simulink model "SADS_UKF"  (R2024b)
settings: Solver=ode15s  StartTime=0.0  StopTime=t_final  RelTol=1e-3
values from neighbouring files (symbols this model uses):
  EA_0 = deg2rad(output(2:4,1))    [telemetry.m]
  g_N = [0 0 -9.81]    [telemetry.m]
  H = [eye(3)  zeros(3,5)]    [telemetry.m]
  J = [1.301  0 0 ... (first row only)    [playground.m]    (also in telemetry.m)
  m_s = 28.542    [playground.m]    (also in telemetry.m)
  omega_0 = output(5:7,1)    [telemetry.m]
  P_0 = diag([1e-6 1e-6 1e-6 1e-6 1e-6 1e-6 1e-6 1e-6])    [telemetry.m]
  process_PSD = (process_variance^2)*T_s    (= 1e-12)    [telemetry.m]
  Q = diag([5e-5 5e-5 5e-5 4e-11 4e-11 4e-11 4e-11 4e-13])    [telemetry.m]
  q_0 = eul2quat(EA_0',"XYZ")'    [telemetry.m]
  R = diag([0.005 0.005 0.003].^2)    [telemetry.m]
  r_0 = [-0.003 0.006 -0.005]'    [telemetry.m]
  sample_time = 1/sample_rate    (= 0.04)    [telemetry.m]
  sensor_PSD = noise_power^2    (= 2.74155703361e-09)    [telemetry.m]
  x_0 = [omega_0; q_0; -0.001]    [telemetry.m]
libraries: simulink x6, sharedtransform x2, simulink_extras x1
settings Model: Creator=camer  LastModifiedBy=camer

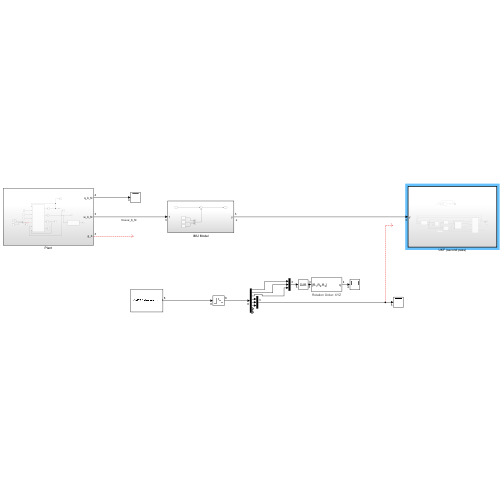
[thumbnail: Simulink's stored preview of the top-level diagram]
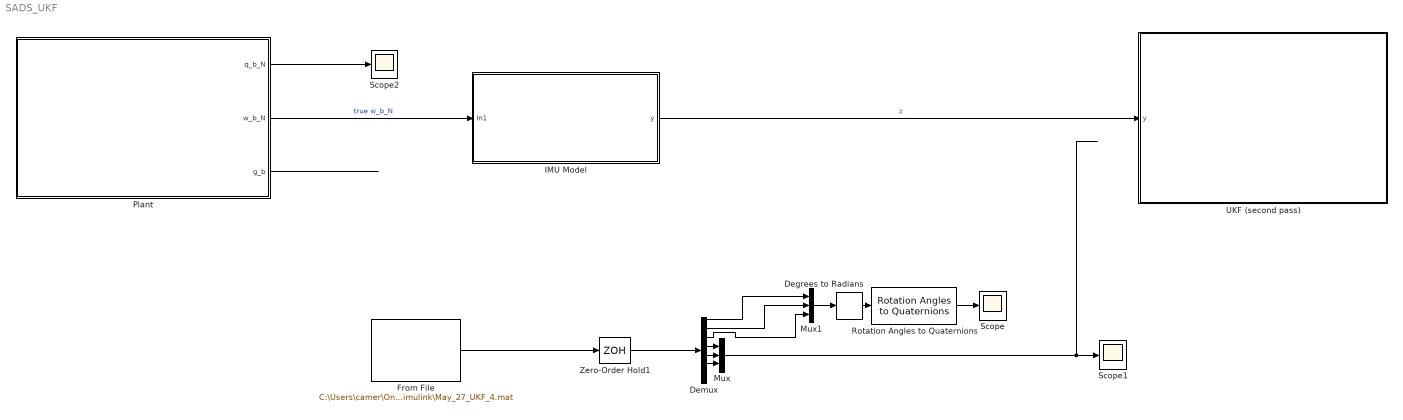
== system SADS_UKF ==
  Degrees to Radians : simulink_extras/Transformations/Degrees to Radians
  Demux : Demux  Outputs=8
  From File : FromFile  FileName=C:\Users\camer\OneDrive\Desktop\SADS Balance\export_for_simulink\May_27_UKF_4.mat  SampleTime=0  InterpolationWithinTimeRange=Zero order hold
  IMU Model : Subsystem
  Mux : Mux  Inputs=3
  Mux1 : Mux  Inputs=3
  Plant : Subsystem
  Rotation Angles to Quaternions : sharedtransform/Rotation Angles to Quaternions  rotationOrder=XYZ  aMode=aMode
  Scope : Scope
  Scope1 : Scope
  Scope2 : Scope
  UKF (second pass) : Subsystem  TreatAsAtomicUnit=on
  Zero-Order Hold1 : ZeroOrderHold  SampleTime=sample_time
  wires:
  Plant/2(w_b_N) -> IMU Model/1(In1)  "true w_b_N"
  Plant/3(g_b) -> ?
  Plant/1(q_b_N) -> Scope2/1
  IMU Model/1(y) -> UKF (second pass)/1(y)  "z"
  Mux/1 -> Scope1/1
  From File/1 -> Zero-Order Hold1/1
  Zero-Order Hold1/1 -> Demux/1
  Demux/4 -> Mux/1
  Demux/5 -> Mux/2
  Demux/6 -> Mux/3
  Demux/1 -> Mux1/1
  Demux/2 -> Mux1/2
  Demux/3 -> Mux1/3
  Mux1/1 -> Degrees to Radians/1
  Degrees to Radians/1 -> Rotation Angles to Quaternions/1
  Rotation Angles to Quaternions/1 -> Scope/1

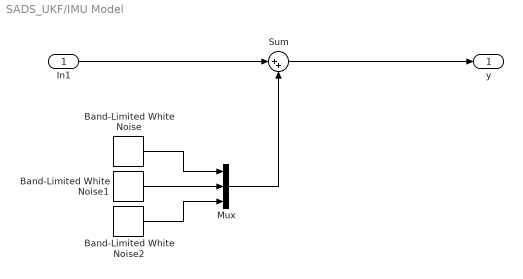
== system SADS_UKF/IMU Model ==
  In1 : Inport
  Band-Limited White Noise : simulink/Sources/Band-Limited White Noise  Cov=[sensor_PSD]  Ts=sample_time  seed=[23341]
  Band-Limited White Noise1 : simulink/Sources/Band-Limited White Noise  Cov=[sensor_PSD]  Ts=sample_time  seed=[23141]
  Band-Limited White Noise2 : simulink/Sources/Band-Limited White Noise  Cov=[sensor_PSD]  Ts=sample_time  seed=[35163]
  Mux : Mux  Inputs=3
  Sum : Sum  Inputs=|++
  y : Outport
  wires:
  Band-Limited White Noise1/1 -> Mux/2
  Band-Limited White Noise/1 -> Mux/1
  Band-Limited White Noise2/1 -> Mux/3
  In1/1 -> Sum/1
  Mux/1 -> Sum/2
  Sum/1 -> y/1

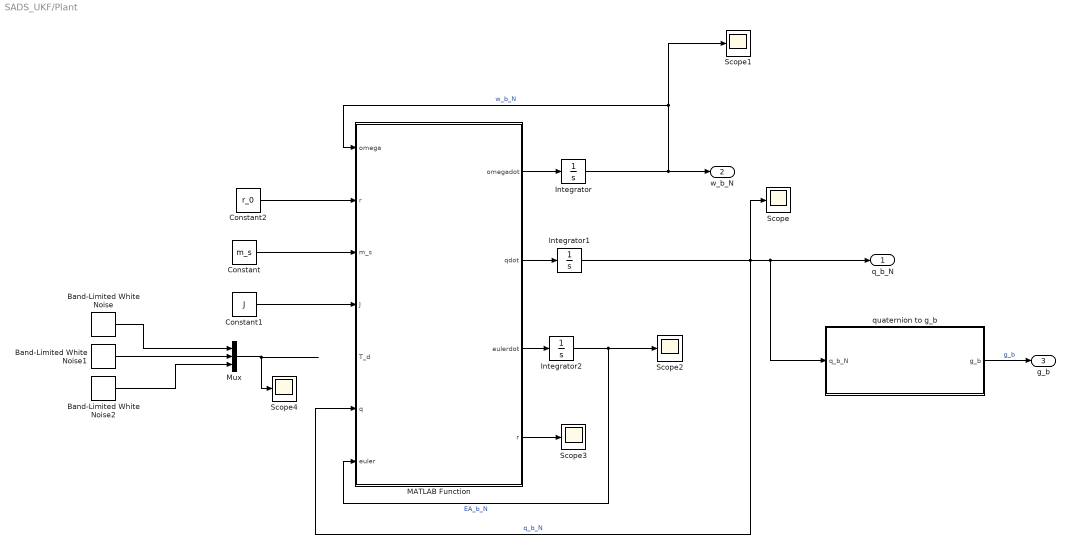
== system SADS_UKF/Plant ==
  Band-Limited White Noise : simulink/Sources/Band-Limited White Noise  Cov=[process_PSD]  Ts=0.1  seed=[23341]
  Band-Limited White Noise1 : simulink/Sources/Band-Limited White Noise  Cov=[process_PSD]  Ts=0.1  seed=[56123]
  Band-Limited White Noise2 : simulink/Sources/Band-Limited White Noise  Cov=[process_PSD]  Ts=0.1  seed=[31256]
  Constant : Constant  Value=m_s
  Constant1 : Constant  Value=J
  Constant2 : Constant  Value=r_0
  Integrator : Integrator  InitialCondition=omega_0
  Integrator1 : Integrator  InitialCondition=q_0
  Integrator2 : Integrator  InitialCondition=EA_0
  MATLAB Function : MATLAB Function  TreatAsAtomicUnit=on
  Mux : Mux  Inputs=3
  Scope{,1..4} (5 alike) : Scope
  quaternion to g_b : Subsystem
  q_b_N : Outport
  w_b_N : Outport  Port=2
  g_b : Outport  Port=3
  wires:
  MATLAB Function/4(r) -> Scope3/1
  Integrator/1 -> Scope1/1, MATLAB Function/1(omega), w_b_N/1  "w_b_N"
  Constant1/1 -> MATLAB Function/4(J)
  Constant2/1 -> MATLAB Function/2("r ")
  Constant/1 -> MATLAB Function/3(m_s)
  Integrator1/1 -> Scope/1, quaternion to g_b/1(q_b_N), q_b_N/1, MATLAB Function/6(q)  "q_b_N"
  MATLAB Function/2(qdot) -> Integrator1/1
  MATLAB Function/1(omegadot) -> Integrator/1
  quaternion to g_b/1(g_b) -> g_b/1  "g_b"
  MATLAB Function/3(eulerdot) -> Integrator2/1
  Integrator2/1 -> Scope2/1, MATLAB Function/7(euler)  "EA_b_N"
  Band-Limited White Noise/1 -> Mux/1
  Band-Limited White Noise1/1 -> Mux/2
  Band-Limited White Noise2/1 -> Mux/3
  Mux/1 -> Scope4/1

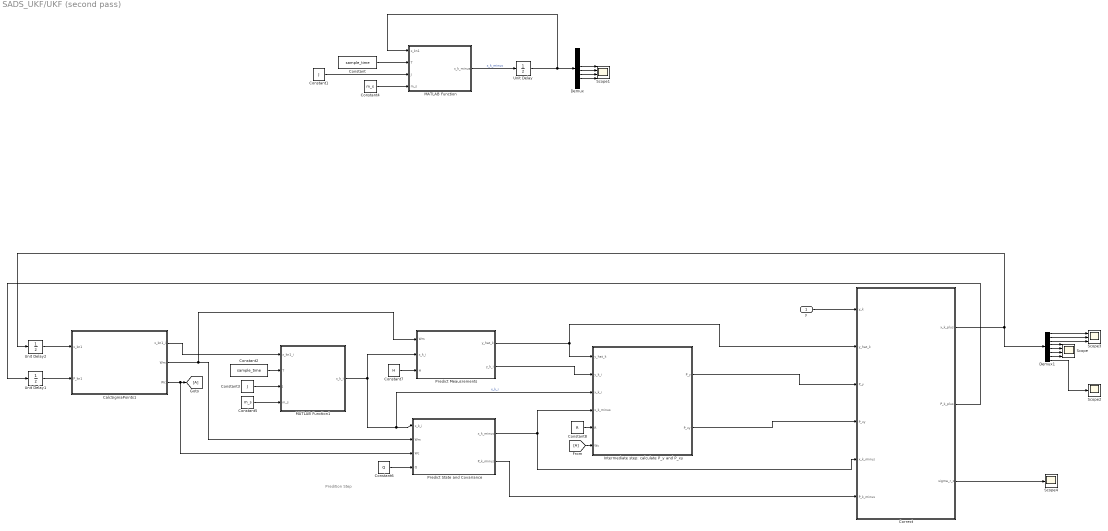
== system SADS_UKF/UKF (second pass) ==
  note: Predition Step
  y : Inport
  CalcSigmaPoints1 : MATLAB Function  TreatAsAtomicUnit=on
  Constant : Constant  Value=sample_time
  Constant1 : Constant  Value=J
  Constant2 : Constant  Value=sample_time
  Constant3 : Constant  Value=J
  Constant4 : Constant  Value=m_s
  Constant5 : Constant  Value=m_s
  Constant6 : Constant  Value=Q
  Constant7 : Constant  Value=H
  Constant8 : Constant  Value=R
  Correct : MATLAB Function  TreatAsAtomicUnit=on
  Demux : Demux  Outputs=8
  Demux1 : Demux  Outputs=8
  From : From
  Goto : Goto
  Intermediate step: calculate P_y and P_xy : MATLAB Function  TreatAsAtomicUnit=on
  MATLAB Function : MATLAB Function  TreatAsAtomicUnit=on
  MATLAB Function1 : MATLAB Function  TreatAsAtomicUnit=on
  Predict Meausrements : MATLAB Function  TreatAsAtomicUnit=on
  Predict State and Covariance : MATLAB Function  TreatAsAtomicUnit=on
  Scope : Scope  NumInputPorts=4
  Scope1 : Scope  NumInputPorts=4
  Scope2 : Scope
  Scope3 : Scope  NumInputPorts=3
  Scope4 : Scope
  Unit Delay : UnitDelay  InitialCondition=x_0  SampleTime=sample_time  HasFrameUpgradeWarning=on
  Unit Delay1 : UnitDelay  InitialCondition=P_0  SampleTime=sample_time  HasFrameUpgradeWarning=on
  Unit Delay2 : UnitDelay  InitialCondition=x_0  SampleTime=sample_time  HasFrameUpgradeWarning=on
  wires:
  MATLAB Function/1(x_k_minus) -> Unit Delay/1  "x_k_minus"
  Constant/1 -> MATLAB Function/2(T)
  Unit Delay/1 -> Demux/1, MATLAB Function/1(x_kn1)
  Constant1/1 -> MATLAB Function/3(J)
  CalcSigmaPoints1/1(x_kn1_i) -> MATLAB Function1/1(x_kn1_i)
  Constant3/1 -> MATLAB Function1/3(J)
  Constant2/1 -> MATLAB Function1/2(T)
  MATLAB Function1/1(x_k_i) -> Intermediate step: calculate P_y and P_xy/3(x_k_i), Predict State and Covariance/1(x_k_i), Predict Meausrements/2(x_k_i)  "x_k_i"
  Constant6/1 -> Predict State and Covariance/4(Q)
  Predict State and Covariance/1(x_k_minus) -> Intermediate step: calculate P_y and P_xy/4(x_k_minus), Correct/5(x_k_minus)
  Predict Meausrements/1(y_hat_k) -> Intermediate step: calculate P_y and P_xy/1(y_hat_k), Correct/2(y_hat_k)
  Predict State and Covariance/2(P_k_minus) -> Correct/6(P_k_minus)
  Constant7/1 -> Predict Meausrements/3(H)
  Predict Meausrements/2(y_k_i) -> Intermediate step: calculate P_y and P_xy/2(y_k_i)
  Constant8/1 -> Intermediate step: calculate P_y and P_xy/5(R)
  y/1 -> Correct/1(y_k)
  Intermediate step: calculate P_y and P_xy/1(P_y) -> Correct/3(P_y)
  Intermediate step: calculate P_y and P_xy/2(P_xy) -> Correct/4(P_xy)
  Correct/2(P_k_plus) -> Unit Delay1/1
  Correct/1(x_k_plus) -> Demux1/1, Unit Delay2/1
  Unit Delay1/1 -> CalcSigmaPoints1/2(P_kn1)
  Unit Delay2/1 -> CalcSigmaPoints1/1(x_kn1)
  CalcSigmaPoints1/2(Wm) -> Predict State and Covariance/2(Wm), Predict Meausrements/1(Wm)
  CalcSigmaPoints1/3(Wc) -> Goto/1, Predict State and Covariance/3(Wc)
  From/1 -> Intermediate step: calculate P_y and P_xy/6(Wc)
  Constant4/1 -> MATLAB Function/4(m_s)
  Demux/4 -> Scope1/1
  Demux/5 -> Scope1/2
  Demux/6 -> Scope1/3
  Demux/7 -> Scope1/4
  Demux1/5 -> Scope/2
  Demux1/4 -> Scope/1
  Demux1/6 -> Scope/3
  Demux1/7 -> Scope/4
  Constant5/1 -> MATLAB Function1/4(m_s)
  Demux1/8 -> Scope2/1
  Demux1/1 -> Scope3/1
  Demux1/2 -> Scope3/2
  Demux1/3 -> Scope3/3
  Correct/3(sigma_r_z) -> Scope4/1

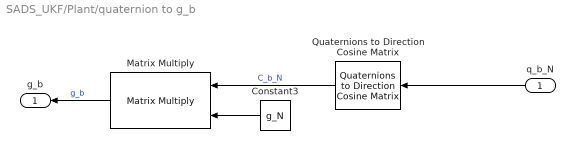
== system SADS_UKF/Plant/quaternion to g_b ==
  q_b_N : Inport
  Constant3 : Constant  Value=g_N
  Matrix Multiply : Product  Multiplication=Matrix(*)
  Quaternions to Direction Cosine Matrix : sharedtransform/Quaternions to  Direction Cosine Matrix  aMode=aMode
  g_b : Outport
  wires:
  Constant3/1 -> Matrix Multiply/2
  Quaternions to Direction Cosine Matrix/1 -> Matrix Multiply/1  "C_b_N"
  q_b_N/1 -> Quaternions to Direction Cosine Matrix/1
  Matrix Multiply/1 -> g_b/1  "g_b"

== matlab function SADS_UKF/UKF (second pass)/Predict State and Covariance ==
  data: x_k_i input; Wm input; Wc input; x_k_minus output; P_k_minus output; Q input
function [x_k_minus,P_k_minus] = predict_state_and_covariance(x_k_i,Wm,Wc,Q)

x_k_minus = x_k_i * Wm;  % weighted mean  (matrix‑vector product)
x_k_minus(4:7) = x_k_minus(4:7)./norm(x_k_minus(4:7));

P_k_minus = (x_k_i - x_k_minus)*diag(Wc) * (x_k_i - x_k_minus)'+ Q;

== matlab function SADS_UKF/Plant/MATLAB Function ==
  data: omega input; r input; m_s input; J input; T_d input; omegadot output; q input; qdot output; eulerdot output; r output; euler input
function [omegadot, qdot,eulerdot,r] = fcn(omega,r,m_s,J,T_d,q,euler)
% Equations of motion developed in the work of Chesi.

g = 9.81; % 

% Gravity vector in body-frame
C_N_b = [2*q(1)^2-1+2*q(2)^2 2*q(2)*q(3)-2*q(1)*q(4) 2*q(2)*q(4)+2*q(1)*q(3);
       2*q(2)*q(3)+2*q(1)*q(4) 2*q(1)^2-1+2*q(3)^2 2*q(3)*q(4)-2*q(1)*q(2);
       2*q(2)*q(4)-2*q(1)*q(3) 2*q(3)*q(4)+2*q(1)*q(2) 2*q(1)^2-1+2*q(4)^2];

g_b = C_N_b' * [0; 0; -g];

u = [1 0 0; % column vectors that each mass slides along
     0 1 0;
     0 0 1];

r_cross_g = [-r(3)*g_b(2) + r(2)*g_b(3);
              r(3)*g_b(1) - r(1)*g_b(3);
             -r(2)*g_b(1) + r(1)*g_b(2);];

r_cross_g = [-r(3)*g_b(2);
              r(3)*g_b(1);
               0];


% Equations of Motion
omegadot=J\(-cross(omega,J*omega)+(m_s*r_cross_g)+T_d);

% Quaternion rates
qdot = 0.5*[0 -omega(1) -omega(2) -omega(3);
             omega(1) 0 omega(3) -omega(2);
             omega(2) -omega(3) 0 omega(1);
             omega(3) omega(2) -omega(1) 0]*q;

% Euler rates
Phi = euler(1);
Theta = euler(2);
Psi = euler(3);

matrix = (1/cos(Theta)).*[cos(Theta) sin(Phi)*sin(Theta)  cos(Phi)*sin(Theta);
                              0          cos(Phi)*cos(Theta) -sin(Phi)*cos(Theta);
                              0          sin(Phi)             cos(Phi)];

product = matrix * omega;

dPhi = product(1);
dTheta = product(2);
dPsi = product(3);

eulerdot = [dPhi dTheta dPsi]';

== matlab function SADS_UKF/UKF (second pass)/CalcSigmaPoints1 ==
  data: x_kn1 input; x_kn1_i output; P_kn1 input; Wm output; Wc output
function [x_kn1_i,Wm,Wc] = calc_sigma_points(x_kn1, P_kn1)

n = size(x_kn1,1);

alpha   = 1e-3;         % small, positive
kappa   = 0;            % usually 0
beta    = 2;            % optimal for Gaussian
lambda  = alpha^2*(n+kappa) - n;

[root,~] = chol((n+lambda)*P_kn1,'lower');

x_kn1_i = zeros(n,2*n + 1);
x_kn1_i(:,1) = x_kn1; % central point

for i = 1:n
    x_kn1_i(:,i+1)   = x_kn1 + root(:,i);
    x_kn1_i(:,i+1+n) = x_kn1 - root(:,i);
end
      

Wm      = 0.5 /(n+lambda) * ones(2*n+1,1);
Wc      = Wm;
Wm(1)   = lambda/(n+lambda);
Wc(1)   = Wm(1) + (1-alpha^2+beta);

== matlab function SADS_UKF/UKF (second pass)/Correct ==
  data: y_k input; y_hat_k input; P_y input; P_xy input; x_k_minus input; x_k_plus output; P_k_minus input; P_k_plus output; sigma_r_z output
function [x_k_plus,P_k_plus,sigma_r_z] = correct(y_k, y_hat_k, P_y,P_xy,x_k_minus,P_k_minus)

K = P_xy/P_y;


x_k_plus = x_k_minus + K*(y_k-y_hat_k);
x_k_plus(4:7) = x_k_plus(4:7)./norm(x_k_plus(4:7));
P_k_plus = P_k_minus - K*P_y*K';

sigma_r_z = sqrt(P_k_plus(end,end));

== matlab function SADS_UKF/UKF (second pass)/Intermediate step: calculate P_y and P_xy ==
  data: y_hat_k input; y_k_i input; P_y output; x_k_i input; x_k_minus input; P_xy output; R input; Wc input
function [P_y,P_xy] = calc_Py_and_Px(y_hat_k,y_k_i,x_k_i,x_k_minus,R,Wc)

diff_y = y_k_i - y_hat_k;
diff_x = x_k_i - x_k_minus;

P_y = diff_y * diag(Wc) * diff_y' + R;
P_xy = diff_x * diag(Wc) * diff_y';

== matlab function SADS_UKF/UKF (second pass)/MATLAB Function ==
  data: x_kn1 input; x_k_minus output; T input; J input; m_s input
function x_k_minus = f(x_kn1,T,J,m_s)
    omega_kn1 = x_kn1(1:3,1);
    eta_kn1 = x_kn1(4);
    eps_kn1 = x_kn1(5:7);
    r_z_kn1 = x_kn1(8);

    % Gravity vector in body-frame
    q = [eta_kn1; eps_kn1;];

    g_b = [2*q(1)^2-1+2*q(2)^2 2*q(2)*q(3)-2*q(1)*q(4) 2*q(2)*q(4)+2*q(1)*q(3);
            2*q(2)*q(3)+2*q(1)*q(4) 2*q(1)^2-1+2*q(3)^2 2*q(3)*q(4)-2*q(1)*q(2);
            2*q(2)*q(4)-2*q(1)*q(3) 2*q(3)*q(4)+2*q(1)*q(2) 2*q(1)^2-1+2*q(4)^2]' * [0; 0; -9.81];

    r_cross_g = [-r_z_kn1*g_b(2);
                  r_z_kn1*g_b(1);
                  0];
        
    omega_kn1_cross = [0           -omega_kn1(3) omega_kn1(2);
                       omega_kn1(3) 0           -omega_kn1(1);
                      -omega_kn1(2) omega_kn1(1) 0];
    
    eps_kn1_cross = [0         -eps_kn1(3) eps_kn1(2);
                     eps_kn1(3) 0         -eps_kn1(1);
                    -eps_kn1(2) eps_kn1(1) 0];
    
    x_k_minus = x_kn1 + T*[inv(J)*(-omega_kn1_cross*J*omega_kn1+m_s*r_cross_g); 
                           -.5*eps_kn1'*omega_kn1;
                            .5*(eta_kn1*eye(3) + eps_kn1_cross)*omega_kn1; 
                            0];

end

== matlab function SADS_UKF/UKF (second pass)/MATLAB Function1 ==
  data: x_kn1_i input; x_k_i output; T input; J input; m_s input
function x_k_i = f(x_kn1_i,T,J,m_s)
    n = size(x_kn1_i,1);
    x_k_i = zeros(n,2*n+1);
    for i = 1:2*n+1
        omega_kn1 = x_kn1_i(1:3,i);
        eta_kn1 = x_kn1_i(4,i);
        eps_kn1 = x_kn1_i(5:7,i);

        q = [eta_kn1; eps_kn1;];
        % Gravity vector in body-frame
        g_b = [2*q(1)^2-1+2*q(2)^2 2*q(2)*q(3)-2*q(1)*q(4) 2*q(2)*q(4)+2*q(1)*q(3);
                2*q(2)*q(3)+2*q(1)*q(4) 2*q(1)^2-1+2*q(3)^2 2*q(3)*q(4)-2*q(1)*q(2);
                2*q(2)*q(4)-2*q(1)*q(3) 2*q(3)*q(4)+2*q(1)*q(2) 2*q(1)^2-1+2*q(4)^2]' * [0; 0; -9.81];

    
        r_z_kn1 = x_kn1_i(8,i);
        
        omega_kn1_cross = [0           -omega_kn1(3) omega_kn1(2);
                           omega_kn1(3) 0           -omega_kn1(1);
                          -omega_kn1(2) omega_kn1(1) 0];
        
        eps_kn1_cross = [0         -eps_kn1(3) eps_kn1(2);
                         eps_kn1(3) 0         -eps_kn1(1);
                        -eps_kn1(2) eps_kn1(1) 0];

        r_cross_g = [-r_z_kn1*g_b(2);
                      r_z_kn1*g_b(1);
                      0];
        
        x_k_i(:,i) = x_kn1_i(:,i) + T*[J\(-omega_kn1_cross*J*omega_kn1 + m_s*r_cross_g); 
                                     -.5*eps_kn1'*omega_kn1
                                      .5*(eta_kn1*eye(3) + eps_kn1_cross)*omega_kn1; 
                                       0];
        
        % normalize the quaternion portion of the state
        x_k_i(4:7,i) = x_k_i(4:7,i)./norm(x_k_i(4:7,i)); 
    end
end

== matlab function SADS_UKF/UKF (second pass)/Predict Meausrements ==
  data: Wm input; y_hat_k output; y_k_i output; x_k_i input; H input
function [y_hat_k,y_k_i]   = predict_measurements(Wm,x_k_i,H)

y_k_i = H * x_k_i;

y_hat_k = y_k_i * Wm;
